simulink model "modellfinal"  (R2019a)
settings: Solver=FixedStepDiscrete  StartTime=0.0  StopTime=20  FixedStep=1  RelTol=1e-3
libraries: simulink x1
settings Model: Creator=Mahesh  LastModifiedBy=Mahesh

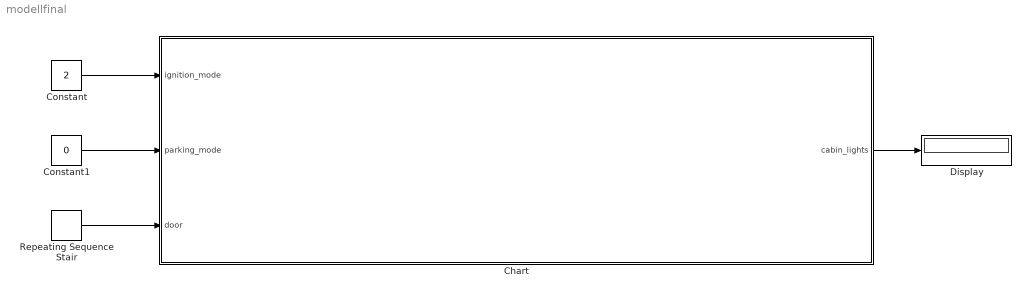
== system modellfinal ==
  Chart : Stateflow chart  BlockKeywords=__PRM__SERIALIZED__DATA__:Stateflow Chart,Stateflow Diagram  TreatAsAtomicUnit=on
  Constant : Constant  Value=2
  Constant1 : Constant  Value=0
  Display : Display
  Repeating Sequence Stair : simulink/Sources/Repeating Sequence Stair  OutValues="[1 1 1  0 0 0 0]"  tsamp=-1  OutMin=[]  OutMax=[]  OutDataTypeStr=double  OutputDataTypeScalingMode=double  OutDataType=fixdt(0,8)  ConRadixGroup=Best Precision: Vector-wise  OutScaling=2^-12
  wires:
  Constant/1 -> Chart/1(ignition_mode)
  Constant1/1 -> Chart/2(parking_mode)
  Chart/1(cabin_lights) -> Display/1
  Repeating Sequence Stair/1 -> Chart/3(door)

== stateflow chart modellfinal/Chart ==
  state end
    en,du:
    cabin_lights=1;
  state start
    en,ex:
    cabin_lights=0;
  (default) -> start
  start -> end [order 2] : [parking_mode==1&&ignition_mode==0]
  end -> start [order 1] : after(5,sec)
  start -> end [order 1] : [door==1]
  end -> start [order 2] : after(3,sec)[door==0]
  data: ignition_mode input; parking_mode input; cabin_lights output; door input
